simulink model "ficom_pr1_ejemplo_canal_simulinkr14"  (Simulink 6.0)
settings: Solver=ode45  StartTime=0.0  StopTime=20.0  RelTol=1e-3
libraries: commnoisgen2 x3, simulink x2, cstblocks x1
settings Model: Creator=fedemp  LastModifiedBy=fedemp  ExtModeAutoUpdateStatusClock=off

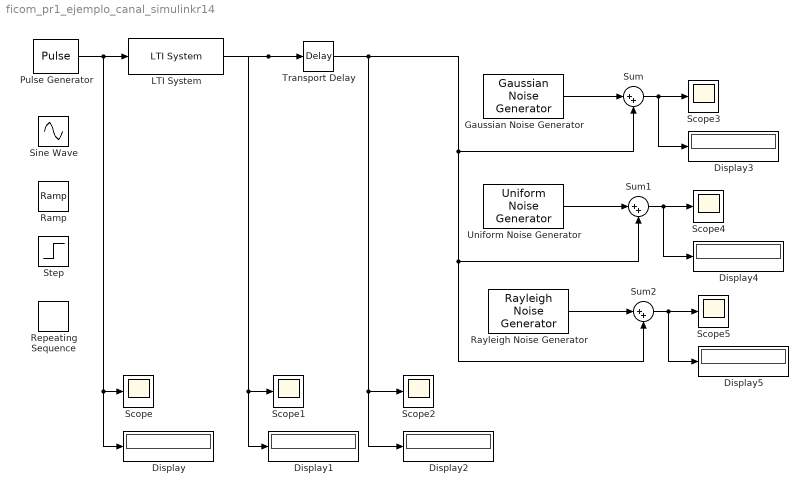
== system ficom_pr1_ejemplo_canal_simulinkr14 ==
  Display{,1..5} (6 alike) : Display
  Gaussian Noise Generator : commnoisgen2/Gaussian Noise Generator  m=0  d=0.6  s=41  Ts=0.01  frameBased=off  sampPerFrame=1  orient=off
  LTI System : cstblocks/LTI System  sys=tf(0.6,[0.5 0.7])  IC=[]
  Pulse Generator : DiscretePulseGenerator  PulseType=Time based  Amplitude=5  Period=2.5  PulseWidth=40
  Ramp : simulink/Sources/Ramp  slope=1  start=0  X0=0
  Rayleigh Noise Generator : commnoisgen2/Rayleigh Noise Generator  alpha=1.3  seed=47  Ts=0.01  frameBased=off  sampPerFrame=1  orient=off
  Repeating Sequence : simulink/Sources/Repeating Sequence  rep_seq_t=[0 2]  rep_seq_y=[0 2]
  Scope{,1..5} (6 alike) : Scope
      Scope2 settings: SaveName=ScopeData2
      Scope3 settings: SaveName=ScopeData3
      Scope4 settings: SaveName=ScopeData4
      Scope5 settings: SaveName=ScopeData5
  Sine Wave : Sin  Amplitude=5  Frequency=0.6  Phase=0.6  SampleTime=0.01
  Step : Step  SampleTime=0
  Sum : Sum  Inputs=|++
  Sum1 : Sum  Inputs=|++
  Sum2 : Sum  Inputs=|++
  Transport Delay : TransportDelay  DelayTime=0.6
  Uniform Noise Generator : commnoisgen2/Uniform Noise Generator  low=0  up=1  seed=31  Ts=0.01  frameBased=off  sampPerFrame=1  orient=off
  wires:
  Pulse Generator/1 -> LTI System/1, Scope/1, Display/1
  LTI System/1 -> Transport Delay/1, Scope1/1, Display1/1
  Transport Delay/1 -> Sum/2, Sum1/2, Sum2/2, Scope2/1, Display2/1
  Gaussian Noise Generator/1 -> Sum/1
  Sum/1 -> Scope3/1, Display3/1
  Uniform Noise Generator/1 -> Sum1/1
  Sum1/1 -> Scope4/1, Display4/1
  Rayleigh Noise Generator/1 -> Sum2/1
  Sum2/1 -> Scope5/1, Display5/1
